simulink model "CLSfixedExample3"  (R2025b)
settings: Solver=FixedStepAuto  StartTime=0.0  StopTime=10  FixedStep=0.0005  RelTol=1e-3
undefined symbols (not defined in the file): AVI, cfg_length, CV1, CV2, LRI, pNode_length, pPath_length, PVARP, stepsize, URI, VRP
libraries: Libs x8, Libs_unified x3
(part 1 of 2)
settings Model: SimulationMode=accelerator  Creator=ball907  LastModifiedBy=rfen801
settings SolverCC: AutoInsertRateTranBlk=on
settings OptimizationCC: DefaultParameterBehavior=Inlined
settings ModelReferenceCC: EnableRefExpFcnMdlSchedulingChecks=on
settings RTWCC: Toolchain=Simulink Real-Time Toolchain  BuildConfiguration=Faster Runs  CodeExecutionProfiling=on

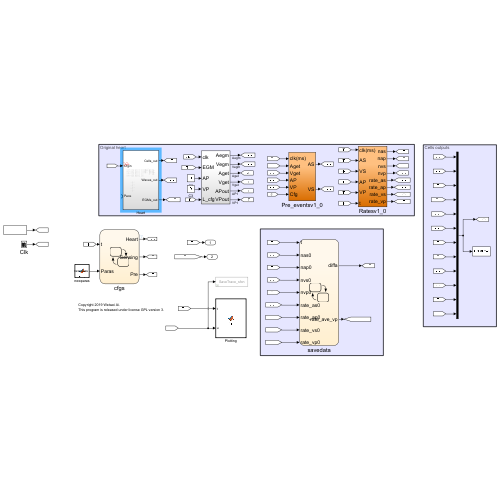
[thumbnail: Simulink's stored preview of the top-level diagram]
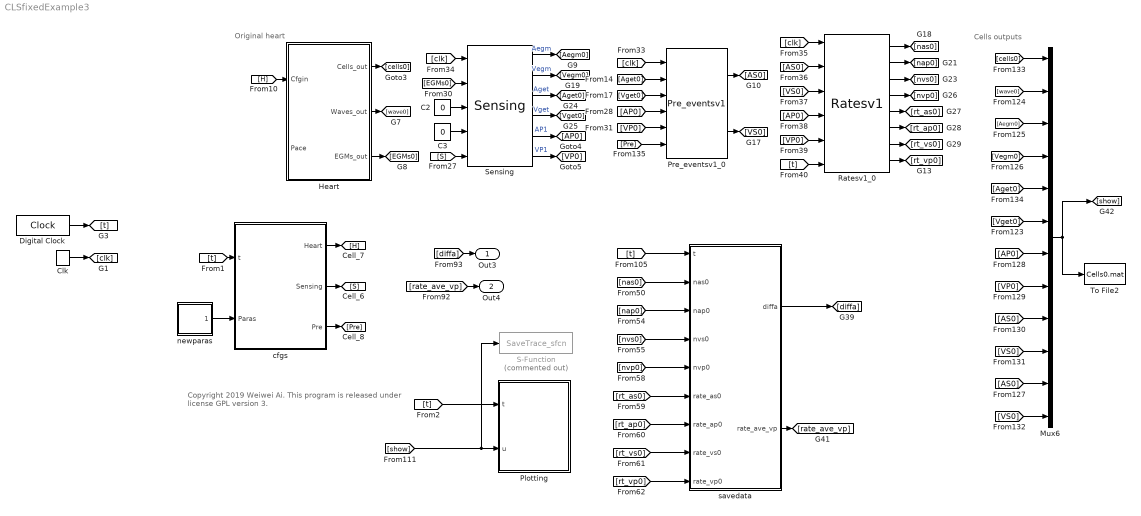
== system CLSfixedExample3 ==
  note: Cells outputs
  note: Copyright 2019 Weiwei Ai.
      | This program is released under license GPL version 3.
  note: Original heart
  C2 : Constant  Value=0
  C3 : Constant  Value=0
  Clk : DiscretePulseGenerator  PulseType=Time based  Period=1  PulseWidth=50
  Digital Clock : DigitalClock  SampleTime=stepsize
  Heart : Subsystem
  Mux6 : Mux  Inputs=12
  Plotting : MATLAB Function  TreatAsAtomicUnit=on  SystemSampleTime=stepsize*5
  Pre_eventsv1_0 : Libs_unified/Pre_eventsv1  SystemSampleTime=-1  VariantActivationTime=update diagram  EmptyChoice=off  PassThrough=off  PassThroughVariantControl=(default)  EmptyChoiceVariantControl=(default)  AllowFlexibleInterface=on  Latency=0  AutoFrameSizeCalculation=off
  Ratesv1_0 : Libs_unified/Ratesv1  SystemSampleTime=-1  VariantActivationTime=update diagram  EmptyChoice=off  PassThrough=off  PassThroughVariantControl=(default)  EmptyChoiceVariantControl=(default)  AllowFlexibleInterface=on  Latency=0  AutoFrameSizeCalculation=off
  S-Function : S-Function  Commented=on  FunctionName=SaveTrace_sfcn  Parameters=1  SFunctionDeploymentMode=off  EnableBusSupport=off
  Sensing : Libs_unified/Sensing  SystemSampleTime=-1  VariantActivationTime=update diagram  EmptyChoice=off  PassThrough=off  PassThroughVariantControl=(default)  EmptyChoiceVariantControl=(default)  AllowFlexibleInterface=on  Latency=0  AutoFrameSizeCalculation=off
  To File2 : ToFile  Filename=Cells0.mat  MatrixName=cells
      settings: Decimation=2
  cfgs : Stateflow chart  TreatAsAtomicUnit=on
  newparas : MATLAB Function  TreatAsAtomicUnit=on
  savedata : Stateflow chart  TreatAsAtomicUnit=on
  Out3 : Outport
  Out4 : Outport  Port=2
  wires:
  Sensing/6 -> [VP0]  "VP1"
  [VS0] -> Mux6/10
  [VS0] -> Ratesv1_0/3
  Pre_eventsv1_0/1 -> [AS0]
  [nap0] -> savedata/3(nap0)
  [VP0] -> Pre_eventsv1_0/5
  [AS0] -> Mux6/11
  Sensing/3 -> [Aget0]  "Aget"
  [rt_ap0] -> savedata/7(rate_ap0)
  C3/1 -> Sensing/4
  [AS0] -> Mux6/9
  Sensing/1 -> [Aegm0]  "Aegm"
  Ratesv1_0/4 -> [nvp0]
  [t] -> savedata/1(t)
  savedata/1(diffa) -> [diffa]
  Heart/3(EGMs_out) -> [EGMs0]
  [cells0] -> Mux6/1
  Pre_eventsv1_0/2 -> [VS0]
  Sensing/4 -> [Vget0]  "Vget"
  Ratesv1_0/5 -> [rt_as0]
  Ratesv1_0/3 -> [nvs0]
  [rt_vp0] -> savedata/9(rate_vp0)
  [rt_vs0] -> savedata/8(rate_vs0)
  [Aget0] -> Pre_eventsv1_0/2
  Sensing/5 -> [AP0]  "AP1"
  Ratesv1_0/1 -> [nas0]
  [diffa] -> Out3/1
  Heart/1(Cells_out) -> [cells0]
  Ratesv1_0/2 -> [nap0]
  [VP0] -> Mux6/8
  Mux6/1 -> [show], To File2/1
  [AS0] -> Ratesv1_0/2
  [AP0] -> Mux6/7
  [t] -> Ratesv1_0/6
  [Aegm0] -> Mux6/3
  [nvs0] -> savedata/4(nvs0)
  [Vget0] -> Mux6/6
  [rt_as0] -> savedata/6(rate_as0)
  [VS0] -> Mux6/12
  [AP0] -> Ratesv1_0/4
  Heart/2(Waves_out) -> [wave0]
  [clk] -> Ratesv1_0/1
  [clk] -> Pre_eventsv1_0/1
  [Pre] -> Pre_eventsv1_0/6
  [Vget0] -> Pre_eventsv1_0/3
  [wave0] -> Mux6/2
  [VP0] -> Ratesv1_0/5
  [AP0] -> Pre_eventsv1_0/4
  savedata/2(rate_ave_vp) -> [rate_ave_vp]
  C2/1 -> Sensing/3
  [S] -> Sensing/5
  [rate_ave_vp] -> Out4/1
  Ratesv1_0/7 -> [rt_vs0]
  [Vegm0] -> Mux6/4
  [clk] -> Sensing/1
  Ratesv1_0/8 -> [rt_vp0]
  [Aget0] -> Mux6/5
  ? -> ?
  [nas0] -> savedata/2(nas0)
  [EGMs0] -> Sensing/2
  Sensing/2 -> [Vegm0]  "Vegm"
  Ratesv1_0/6 -> [rt_ap0]
  [nvp0] -> savedata/5(nvp0)
  cfgs/2(Sensing) -> [S]
  cfgs/3(Pre) -> [Pre]
  newparas/1(newparas) -> cfgs/2(Paras)
  cfgs/1(Heart) -> [H]
  [t] -> cfgs/1(t)
  Digital Clock/1 -> [t]
  Clk/1 -> [clk]
  [show] -> S-Function/1, Plotting/2(u)
  [t] -> Plotting/1(t)
  [H] -> Heart/1(Cfgin)

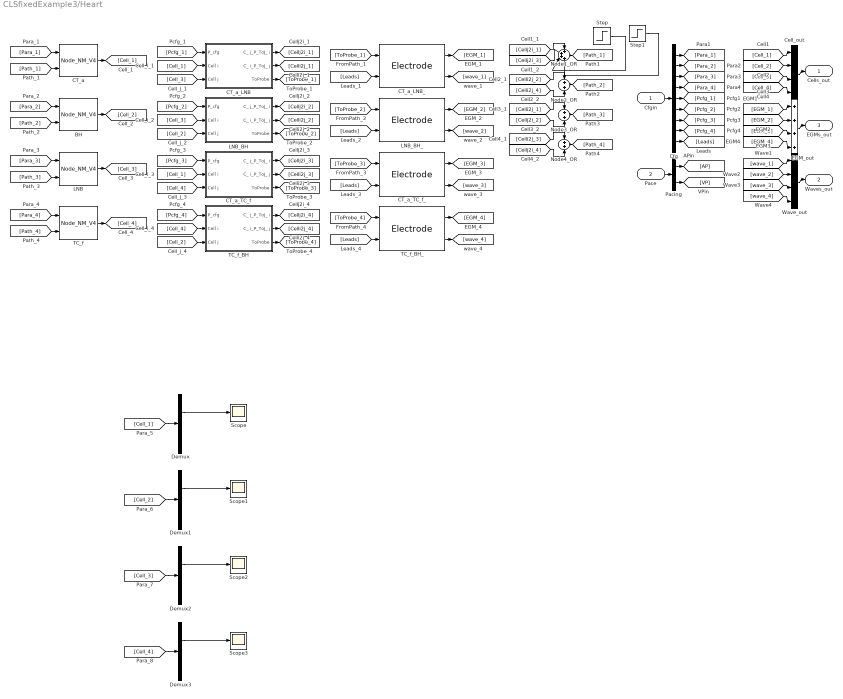
== system CLSfixedExample3/Heart ==
  Cfgin : Inport
  Pace : Inport  Port=2
  BH : Libs/Node_NM_V4  SystemSampleTime=-1  VariantActivationTime=update diagram  EmptyChoice=off  PassThrough=off  PassThroughVariantControl=(default)  EmptyChoiceVariantControl=(default)  AllowFlexibleInterface=on  Latency=0  AutoFrameSizeCalculation=off
  CT_a : Libs/Node_NM_V4  SystemSampleTime=-1  VariantActivationTime=update diagram  EmptyChoice=off  PassThrough=off  PassThroughVariantControl=(default)  EmptyChoiceVariantControl=(default)  AllowFlexibleInterface=on  Latency=0  AutoFrameSizeCalculation=off
  CT_a_LNB : Subsystem  AncestorBlock=Libs/Path_V3
  CT_a_LNB_ : Libs/Electrode  SystemSampleTime=-1  VariantActivationTime=update diagram  EmptyChoice=off  PassThrough=off  PassThroughVariantControl=(default)  EmptyChoiceVariantControl=(default)  AllowFlexibleInterface=on  Latency=0  AutoFrameSizeCalculation=off
  CT_a_TC_f : Subsystem  AncestorBlock=Libs/Path_V3
  CT_a_TC_f_ : Libs/Electrode  SystemSampleTime=-1  VariantActivationTime=update diagram  EmptyChoice=off  PassThrough=off  PassThroughVariantControl=(default)  EmptyChoiceVariantControl=(default)  AllowFlexibleInterface=on  Latency=0  AutoFrameSizeCalculation=off
  Cell_out : Mux
  Cfg : Demux  Outputs=[50,50,50,50,11,11,11,11,28]
  Demux{,1..3} (4 alike) : Demux  Outputs=5
  EGM_out : Sum  Inputs=4
  LNB : Libs/Node_NM_V4  SystemSampleTime=-1  VariantActivationTime=update diagram  EmptyChoice=off  PassThrough=off  PassThroughVariantControl=(default)  EmptyChoiceVariantControl=(default)  AllowFlexibleInterface=on  Latency=0  AutoFrameSizeCalculation=off
  LNB_BH : Subsystem  AncestorBlock=Libs/Path_V3
  LNB_BH_ : Libs/Electrode  SystemSampleTime=-1  VariantActivationTime=update diagram  EmptyChoice=off  PassThrough=off  PassThroughVariantControl=(default)  EmptyChoiceVariantControl=(default)  AllowFlexibleInterface=on  Latency=0  AutoFrameSizeCalculation=off
  Node1_OR : Sum  Inputs=4
  Node2_OR : Sum  Inputs=2
  Node3_OR : Sum  Inputs=2
  Node4_OR : Sum  Inputs=2
  Pacing : Demux  Outputs=2
  Scope{,1..3} (4 alike) : Scope
      Scope settings: ActiveDisplayYMinimum=-14.055953139718371  ActiveDisplayYMaximum=126.50357825746536
      Scope1 settings: ActiveDisplayYMinimum=-16.387499999999996  ActiveDisplayYMaximum=147.48749999999998
      Scope2 settings: ActiveDisplayYMinimum=-16.387499999999996  ActiveDisplayYMaximum=147.48749999999998  DataLoggingVariableName=ScopeData2
      Scope3 settings: ActiveDisplayYMinimum=-14.055953139718371  ActiveDisplayYMaximum=126.50357825746536  DataLoggingVariableName=ScopeData3
  Step : Step  Time=3.32  After=120  SampleTime=0
  Step1 : Step  Time=3.36  After=-120  SampleTime=0
  TC_f : Libs/Node_NM_V4  SystemSampleTime=-1  VariantActivationTime=update diagram  EmptyChoice=off  PassThrough=off  PassThroughVariantControl=(default)  EmptyChoiceVariantControl=(default)  AllowFlexibleInterface=on  Latency=0  AutoFrameSizeCalculation=off
  TC_f_BH : Subsystem  AncestorBlock=Libs/Path_V3
  TC_f_BH_ : Libs/Electrode  SystemSampleTime=-1  VariantActivationTime=update diagram  EmptyChoice=off  PassThrough=off  PassThroughVariantControl=(default)  EmptyChoiceVariantControl=(default)  AllowFlexibleInterface=on  Latency=0  AutoFrameSizeCalculation=off
  Wave_out : Mux
  Cells_out : Outport
  Waves_out : Outport  Port=2
  EGMs_out : Outport  Port=3
  wires:
  Demux1/2 -> Scope1/1
  [Cell_1] -> Demux/1
  [Cell_2] -> Demux1/1
  Demux/2 -> Scope/1
  [Cell_4] -> Demux3/1
  Demux3/2 -> Scope3/1
  [Cell_3] -> Demux2/1
  Demux2/2 -> Scope2/1
  Step1/1 -> Node1_OR/4
  Step/1 -> Node1_OR/3
  [wave_4] -> Wave_out/4
  [wave_3] -> Wave_out/3
  [wave_2] -> Wave_out/2
  [wave_1] -> Wave_out/1
  [EGM_4] -> EGM_out/4
  [EGM_3] -> EGM_out/3
  [EGM_2] -> EGM_out/2
  [EGM_1] -> EGM_out/1
  [Cell_4] -> Cell_out/4
  [Cell_3] -> Cell_out/3
  [Cell_2] -> Cell_out/2
  [Cell_1] -> Cell_out/1
  Wave_out/1 -> Waves_out/1
  EGM_out/1 -> EGMs_out/1
  Cell_out/1 -> Cells_out/1
  Pacing/2 -> [VP]
  Pacing/1 -> [AP]
  Cfg/9 -> [Leads]
  Cfg/8 -> [Pcfg_4]
  Cfg/7 -> [Pcfg_3]
  Cfg/6 -> [Pcfg_2]
  Cfg/5 -> [Pcfg_1]
  Cfg/4 -> [Para_4]
  Cfg/3 -> [Para_3]
  Cfg/2 -> [Para_2]
  Cfg/1 -> [Para_1]
  Pace/1 -> Pacing/1
  Cfgin/1 -> Cfg/1
  Node4_OR/1 -> [Path_4]
  [Cellj2i_4] -> Node4_OR/2
  [Celli2j_3] -> Node4_OR/1
  Node3_OR/1 -> [Path_3]
  [Cellj2i_2] -> Node3_OR/2
  [Celli2j_1] -> Node3_OR/1
  Node2_OR/1 -> [Path_2]
  [Celli2j_4] -> Node2_OR/2
  [Celli2j_2] -> Node2_OR/1
  Node1_OR/1 -> [Path_1]
  [Cellj2i_3] -> Node1_OR/2
  [Cellj2i_1] -> Node1_OR/1
  [Leads] -> TC_f_BH_/2
  [ToProbe_4] -> TC_f_BH_/1
  TC_f_BH_/2 -> [wave_4]
  TC_f_BH_/1 -> [EGM_4]
  [Leads] -> CT_a_TC_f_/2
  [ToProbe_3] -> CT_a_TC_f_/1
  CT_a_TC_f_/2 -> [wave_3]
  CT_a_TC_f_/1 -> [EGM_3]
  [Leads] -> LNB_BH_/2
  [ToProbe_2] -> LNB_BH_/1
  LNB_BH_/2 -> [wave_2]
  LNB_BH_/1 -> [EGM_2]
  [Leads] -> CT_a_LNB_/2
  [ToProbe_1] -> CT_a_LNB_/1
  CT_a_LNB_/2 -> [wave_1]
  CT_a_LNB_/1 -> [EGM_1]
  [Cell_2] -> TC_f_BH/3(Cell j)
  [Cell_4] -> TC_f_BH/2(Cell i)
  [Pcfg_4] -> TC_f_BH/1(P_cfg)
  TC_f_BH/3(ToProbe) -> [ToProbe_4]
  TC_f_BH/2(C_ i_P_ToJ_ j) -> [Celli2j_4]
  TC_f_BH/1(C_ j_P_ToJ_ i) -> [Cellj2i_4]
  [Cell_4] -> CT_a_TC_f/3(Cell j)
  [Cell_1] -> CT_a_TC_f/2(Cell i)
  [Pcfg_3] -> CT_a_TC_f/1(P_cfg)
  CT_a_TC_f/3(ToProbe) -> [ToProbe_3]
  CT_a_TC_f/2(C_ i_P_ToJ_ j) -> [Celli2j_3]
  CT_a_TC_f/1(C_ j_P_ToJ_ i) -> [Cellj2i_3]
  [Cell_2] -> LNB_BH/3(Cell j)
  [Cell_3] -> LNB_BH/2(Cell i)
  [Pcfg_2] -> LNB_BH/1(P_cfg)
  LNB_BH/3(ToProbe) -> [ToProbe_2]
  LNB_BH/2(C_ i_P_ToJ_ j) -> [Celli2j_2]
  LNB_BH/1(C_ j_P_ToJ_ i) -> [Cellj2i_2]
  [Cell_3] -> CT_a_LNB/3(Cell j)
  [Cell_1] -> CT_a_LNB/2(Cell i)
  [Pcfg_1] -> CT_a_LNB/1(P_cfg)
  CT_a_LNB/3(ToProbe) -> [ToProbe_1]
  CT_a_LNB/2(C_ i_P_ToJ_ j) -> [Celli2j_1]
  CT_a_LNB/1(C_ j_P_ToJ_ i) -> [Cellj2i_1]
  [Path_4] -> TC_f/2
  [Para_4] -> TC_f/1
  TC_f/1 -> [Cell_4]
  [Path_3] -> LNB/2
  [Para_3] -> LNB/1
  LNB/1 -> [Cell_3]
  [Path_2] -> BH/2
  [Para_2] -> BH/1
  BH/1 -> [Cell_2]
  [Path_1] -> CT_a/2
  [Para_1] -> CT_a/1
  CT_a/1 -> [Cell_1]

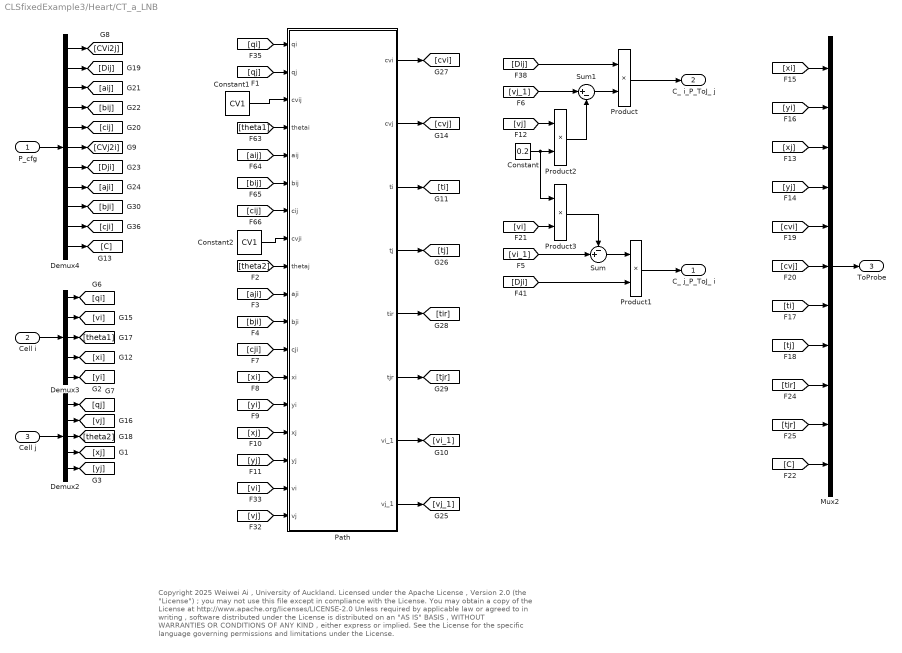
== system CLSfixedExample3/Heart/CT_a_LNB ==
  note: Copyright 2025 Weiwei Ai , University of Auckland.
      | Licensed under the Apache License , Version 2.0 (the "License") ;
      | you may not use this file except in compliance with the License.
      | You may obtain a copy of the License at
      | http://www.apache.org/licenses/LICENSE-2.0
      | Unless required by applicable law or agreed to in writing , software
      | distributed under the License is distributed on an "AS IS" BASIS ,
      | WITHOUT WARRANTIES OR CONDITIONS OF ANY KIND , either express or implied.
      | See the License for the specific language governing permissions and
      | limitations under the License.
  P_cfg : Inport
  Cell i : Inport  Port=2
  Cell j : Inport  Port=3
  Constant : Constant  Value=0.2
  Constant1 : Constant  Value=CV1
  Constant2 : Constant  Value=CV1
  Demux2 : Demux  Outputs=5
  Demux3 : Demux  Outputs=5
  Demux4 : Demux  Outputs=11
  Mux2 : Mux  Inputs=11
  Path : Stateflow chart  TreatAsAtomicUnit=on
  Product{,1..3} (4 alike) : Product  Inputs=**
  Sum : Sum  Inputs=-+|
  Sum1 : Sum  Inputs=|+-
  C_ j_P_ToJ_ i : Outport
  C_ i_P_ToJ_ j : Outport  Port=2
  ToProbe : Outport  Port=3
  wires:
  [vi] -> Product3/2
  [Dji] -> Product1/2
  [vi_1] -> Sum/2
  Product3/1 -> Sum/1
  Sum/1 -> Product1/1
  Constant/1 -> Product2/2, Product3/1
  Product2/1 -> Sum1/2
  [vj] -> Product2/1
  Sum1/1 -> Product/2
  [vj_1] -> Sum1/1
  Mux2/1 -> ToProbe/1
  [C] -> Mux2/11
  [tjr] -> Mux2/10
  [tj] -> Mux2/8
  [ti] -> Mux2/7
  [cvj] -> Mux2/6
  [tir] -> Mux2/9
  [cvi] -> Mux2/5
  [yj] -> Mux2/4
  [xj] -> Mux2/3
  [yi] -> Mux2/2
  [xi] -> Mux2/1
  Path/6(tjr) -> [tjr]
  Path/5(tir) -> [tir]
  Path/4(tj) -> [tj]
  Path/3(ti) -> [ti]
  Path/2(cvj) -> [cvj]
  Path/1(cvi) -> [cvi]
  Path/7(vi_1) -> [vi_1]
  Path/8(vj_1) -> [vj_1]
  [qj] -> Path/2(qj)
  Constant2/1 -> Path/8(cvji)
  [theta2] -> Path/9(thetaj)
  [aji] -> Path/10(aji)
  [bji] -> Path/11(bji)
  [cji] -> Path/12(cji)
  Demux4/6 -> [CVj2i]
  Demux4/7 -> [Dji]
  Demux4/8 -> [aji]
  Demux4/9 -> [bji]
  Demux4/10 -> [cji]
  Demux4/11 -> [C]
  Constant1/1 -> Path/3(cvij)
  [yj] -> Path/16(yj)
  [xj] -> Path/15(xj)
  [yi] -> Path/14(yi)
  [xi] -> Path/13(xi)
  Demux4/1 -> [CVi2j]
  Demux4/5 -> [cij]
  Demux4/4 -> [bij]
  Demux4/3 -> [aij]
  Demux4/2 -> [Dij]
  [cij] -> Path/7(cij)
  [bij] -> Path/6(bij)
  [aij] -> Path/5(aij)
  [theta1] -> Path/4(thetai)
  [Dij] -> Product/1
  Demux2/3 -> [theta2]
  Demux3/3 -> [theta1]
  [vj] -> Path/18(vj)
  Demux2/2 -> [vj]
  [vi] -> Path/17(vi)
  Demux3/2 -> [vi]
  Demux2/5 -> [yj]
  Demux2/4 -> [xj]
  Demux3/5 -> [yi]
  Demux3/4 -> [xi]
  Demux2/1 -> [qj]
  [qi] -> Path/1(qi)
  Demux3/1 -> [qi]
  Product1/1 -> C_ j_P_ToJ_ i/1
  Product/1 -> C_ i_P_ToJ_ j/1
  P_cfg/1 -> Demux4/1
  Cell j/1 -> Demux2/1
  Cell i/1 -> Demux3/1

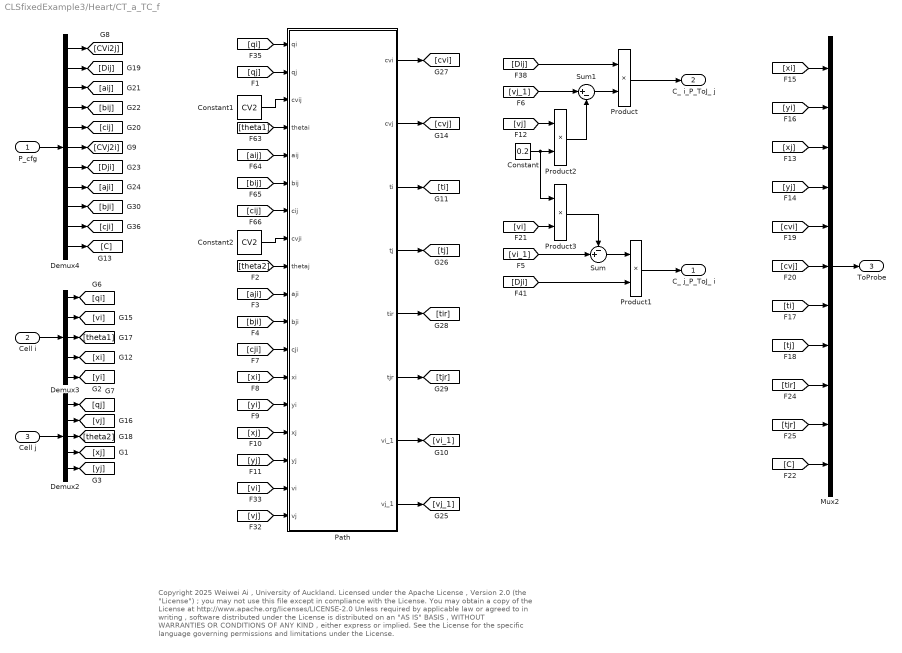
== system CLSfixedExample3/Heart/CT_a_TC_f ==
  note: Copyright 2025 Weiwei Ai , University of Auckland.
      | Licensed under the Apache License , Version 2.0 (the "License") ;
      | you may not use this file except in compliance with the License.
      | You may obtain a copy of the License at
      | http://www.apache.org/licenses/LICENSE-2.0
      | Unless required by applicable law or agreed to in writing , software
      | distributed under the License is distributed on an "AS IS" BASIS ,
      | WITHOUT WARRANTIES OR CONDITIONS OF ANY KIND , either express or implied.
      | See the License for the specific language governing permissions and
      | limitations under the License.
  P_cfg : Inport
  Cell i : Inport  Port=2
  Cell j : Inport  Port=3
  Constant : Constant  Value=0.2
  Constant1 : Constant  Value=CV2
  Constant2 : Constant  Value=CV2
  Demux2 : Demux  Outputs=5
  Demux3 : Demux  Outputs=5
  Demux4 : Demux  Outputs=11
  Mux2 : Mux  Inputs=11
  Path : Stateflow chart  TreatAsAtomicUnit=on
  Product{,1..3} (4 alike) : Product  Inputs=**
  Sum : Sum  Inputs=-+|
  Sum1 : Sum  Inputs=|+-
  C_ j_P_ToJ_ i : Outport
  C_ i_P_ToJ_ j : Outport  Port=2
  ToProbe : Outport  Port=3
  wires:
  [vi] -> Product3/2
  [Dji] -> Product1/2
  [vi_1] -> Sum/2
  Product3/1 -> Sum/1
  Sum/1 -> Product1/1
  Constant/1 -> Product2/2, Product3/1
  Product2/1 -> Sum1/2
  [vj] -> Product2/1
  Sum1/1 -> Product/2
  [vj_1] -> Sum1/1
  Mux2/1 -> ToProbe/1
  [C] -> Mux2/11
  [tjr] -> Mux2/10
  [tj] -> Mux2/8
  [ti] -> Mux2/7
  [cvj] -> Mux2/6
  [tir] -> Mux2/9
  [cvi] -> Mux2/5
  [yj] -> Mux2/4
  [xj] -> Mux2/3
  [yi] -> Mux2/2
  [xi] -> Mux2/1
  Path/6(tjr) -> [tjr]
  Path/5(tir) -> [tir]
  Path/4(tj) -> [tj]
  Path/3(ti) -> [ti]
  Path/2(cvj) -> [cvj]
  Path/1(cvi) -> [cvi]
  Path/7(vi_1) -> [vi_1]
  Path/8(vj_1) -> [vj_1]
  [qj] -> Path/2(qj)
  Constant2/1 -> Path/8(cvji)
  [theta2] -> Path/9(thetaj)
  [aji] -> Path/10(aji)
  [bji] -> Path/11(bji)
  [cji] -> Path/12(cji)
  Demux4/6 -> [CVj2i]
  Demux4/7 -> [Dji]
  Demux4/8 -> [aji]
  Demux4/9 -> [bji]
  Demux4/10 -> [cji]
  Demux4/11 -> [C]
  Constant1/1 -> Path/3(cvij)
  [yj] -> Path/16(yj)
  [xj] -> Path/15(xj)
  [yi] -> Path/14(yi)
  [xi] -> Path/13(xi)
  Demux4/1 -> [CVi2j]
  Demux4/5 -> [cij]
  Demux4/4 -> [bij]
  Demux4/3 -> [aij]
  Demux4/2 -> [Dij]
  [cij] -> Path/7(cij)
  [bij] -> Path/6(bij)
  [aij] -> Path/5(aij)
  [theta1] -> Path/4(thetai)
  [Dij] -> Product/1
  Demux2/3 -> [theta2]
  Demux3/3 -> [theta1]
  [vj] -> Path/18(vj)
  Demux2/2 -> [vj]
  [vi] -> Path/17(vi)
  Demux3/2 -> [vi]
  Demux2/5 -> [yj]
  Demux2/4 -> [xj]
  Demux3/5 -> [yi]
  Demux3/4 -> [xi]
  Demux2/1 -> [qj]
  [qi] -> Path/1(qi)
  Demux3/1 -> [qi]
  Product1/1 -> C_ j_P_ToJ_ i/1
  Product/1 -> C_ i_P_ToJ_ j/1
  P_cfg/1 -> Demux4/1
  Cell j/1 -> Demux2/1
  Cell i/1 -> Demux3/1

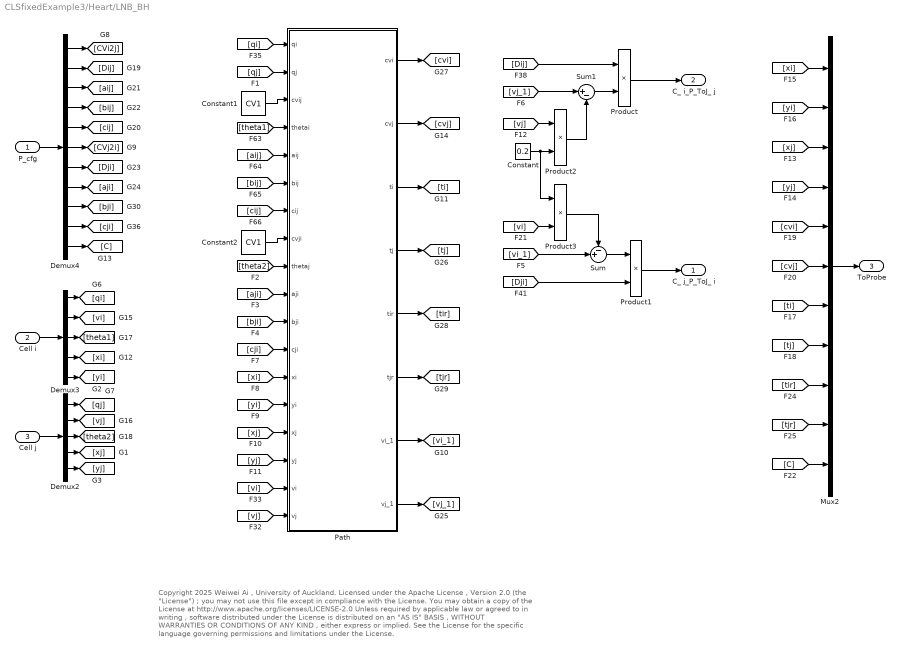
== system CLSfixedExample3/Heart/LNB_BH ==
  note: Copyright 2025 Weiwei Ai , University of Auckland.
      | Licensed under the Apache License , Version 2.0 (the "License") ;
      | you may not use this file except in compliance with the License.
      | You may obtain a copy of the License at
      | http://www.apache.org/licenses/LICENSE-2.0
      | Unless required by applicable law or agreed to in writing , software
      | distributed under the License is distributed on an "AS IS" BASIS ,
      | WITHOUT WARRANTIES OR CONDITIONS OF ANY KIND , either express or implied.
      | See the License for the specific language governing permissions and
      | limitations under the License.
  P_cfg : Inport
  Cell i : Inport  Port=2
  Cell j : Inport  Port=3
  Constant : Constant  Value=0.2
  Constant1 : Constant  Value=CV1
  Constant2 : Constant  Value=CV1
  Demux2 : Demux  Outputs=5
  Demux3 : Demux  Outputs=5
  Demux4 : Demux  Outputs=11
  Mux2 : Mux  Inputs=11
  Path : Stateflow chart  TreatAsAtomicUnit=on
  Product{,1..3} (4 alike) : Product  Inputs=**
  Sum : Sum  Inputs=-+|
  Sum1 : Sum  Inputs=|+-
  C_ j_P_ToJ_ i : Outport
  C_ i_P_ToJ_ j : Outport  Port=2
  ToProbe : Outport  Port=3
  wires:
  [vi] -> Product3/2
  [Dji] -> Product1/2
  [vi_1] -> Sum/2
  Product3/1 -> Sum/1
  Sum/1 -> Product1/1
  Constant/1 -> Product2/2, Product3/1
  Product2/1 -> Sum1/2
  [vj] -> Product2/1
  Sum1/1 -> Product/2
  [vj_1] -> Sum1/1
  Mux2/1 -> ToProbe/1
  [C] -> Mux2/11
  [tjr] -> Mux2/10
  [tj] -> Mux2/8
  [ti] -> Mux2/7
  [cvj] -> Mux2/6
  [tir] -> Mux2/9
  [cvi] -> Mux2/5
  [yj] -> Mux2/4
  [xj] -> Mux2/3
  [yi] -> Mux2/2
  [xi] -> Mux2/1
  Path/6(tjr) -> [tjr]
  Path/5(tir) -> [tir]
  Path/4(tj) -> [tj]
  Path/3(ti) -> [ti]
  Path/2(cvj) -> [cvj]
  Path/1(cvi) -> [cvi]
  Path/7(vi_1) -> [vi_1]
  Path/8(vj_1) -> [vj_1]
  [qj] -> Path/2(qj)
  Constant2/1 -> Path/8(cvji)
  [theta2] -> Path/9(thetaj)
  [aji] -> Path/10(aji)
  [bji] -> Path/11(bji)
  [cji] -> Path/12(cji)
  Demux4/6 -> [CVj2i]
  Demux4/7 -> [Dji]
  Demux4/8 -> [aji]
  Demux4/9 -> [bji]
  Demux4/10 -> [cji]
  Demux4/11 -> [C]
  Constant1/1 -> Path/3(cvij)
  [yj] -> Path/16(yj)
  [xj] -> Path/15(xj)
  [yi] -> Path/14(yi)
  [xi] -> Path/13(xi)
  Demux4/1 -> [CVi2j]
  Demux4/5 -> [cij]
  Demux4/4 -> [bij]
  Demux4/3 -> [aij]
  Demux4/2 -> [Dij]
  [cij] -> Path/7(cij)
  [bij] -> Path/6(bij)
  [aij] -> Path/5(aij)
  [theta1] -> Path/4(thetai)
  [Dij] -> Product/1
  Demux2/3 -> [theta2]
  Demux3/3 -> [theta1]
  [vj] -> Path/18(vj)
  Demux2/2 -> [vj]
  [vi] -> Path/17(vi)
  Demux3/2 -> [vi]
  Demux2/5 -> [yj]
  Demux2/4 -> [xj]
  Demux3/5 -> [yi]
  Demux3/4 -> [xi]
  Demux2/1 -> [qj]
  [qi] -> Path/1(qi)
  Demux3/1 -> [qi]
  Product1/1 -> C_ j_P_ToJ_ i/1
  Product/1 -> C_ i_P_ToJ_ j/1
  P_cfg/1 -> Demux4/1
  Cell j/1 -> Demux2/1
  Cell i/1 -> Demux3/1

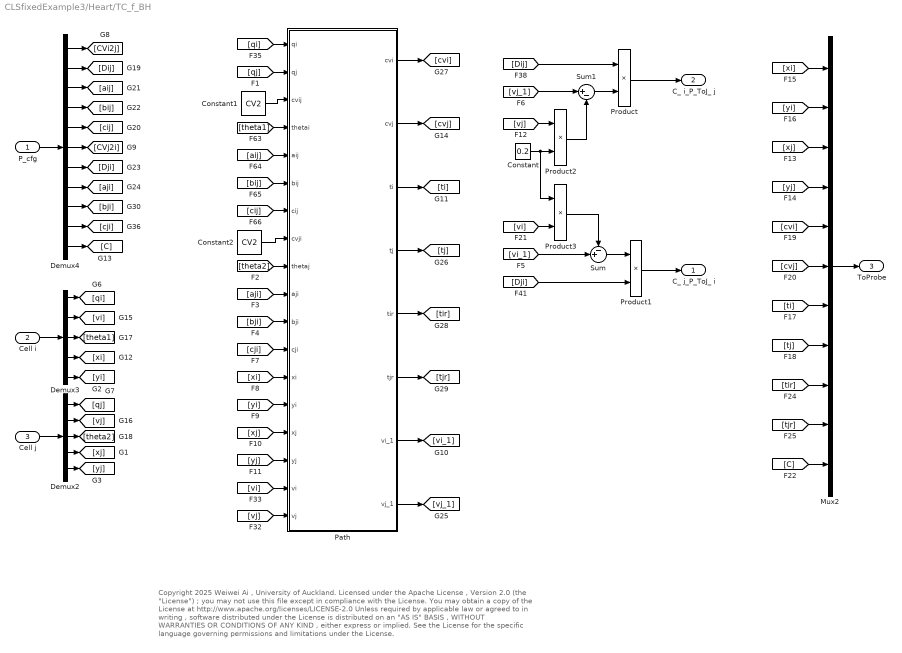
== system CLSfixedExample3/Heart/TC_f_BH ==
  note: Copyright 2025 Weiwei Ai , University of Auckland.
      | Licensed under the Apache License , Version 2.0 (the "License") ;
      | you may not use this file except in compliance with the License.
      | You may obtain a copy of the License at
      | http://www.apache.org/licenses/LICENSE-2.0
      | Unless required by applicable law or agreed to in writing , software
      | distributed under the License is distributed on an "AS IS" BASIS ,
      | WITHOUT WARRANTIES OR CONDITIONS OF ANY KIND , either express or implied.
      | See the License for the specific language governing permissions and
      | limitations under the License.
  P_cfg : Inport
  Cell i : Inport  Port=2
  Cell j : Inport  Port=3
  Constant : Constant  Value=0.2
  Constant1 : Constant  Value=CV2
  Constant2 : Constant  Value=CV2
  Demux2 : Demux  Outputs=5
  Demux3 : Demux  Outputs=5
  Demux4 : Demux  Outputs=11
  Mux2 : Mux  Inputs=11
  Path : Stateflow chart  TreatAsAtomicUnit=on
  Product{,1..3} (4 alike) : Product  Inputs=**
  Sum : Sum  Inputs=-+|
  Sum1 : Sum  Inputs=|+-
  C_ j_P_ToJ_ i : Outport
  C_ i_P_ToJ_ j : Outport  Port=2
  ToProbe : Outport  Port=3
  wires:
  [vi] -> Product3/2
  [Dji] -> Product1/2
  [vi_1] -> Sum/2
  Product3/1 -> Sum/1
  Sum/1 -> Product1/1
  Constant/1 -> Product2/2, Product3/1
  Product2/1 -> Sum1/2
  [vj] -> Product2/1
  Sum1/1 -> Product/2
  [vj_1] -> Sum1/1
  Mux2/1 -> ToProbe/1
  [C] -> Mux2/11
  [tjr] -> Mux2/10
  [tj] -> Mux2/8
  [ti] -> Mux2/7
  [cvj] -> Mux2/6
  [tir] -> Mux2/9
  [cvi] -> Mux2/5
  [yj] -> Mux2/4
  [xj] -> Mux2/3
  [yi] -> Mux2/2
  [xi] -> Mux2/1
  Path/6(tjr) -> [tjr]
  Path/5(tir) -> [tir]
  Path/4(tj) -> [tj]
  Path/3(ti) -> [ti]
  Path/2(cvj) -> [cvj]
  Path/1(cvi) -> [cvi]
  Path/7(vi_1) -> [vi_1]
  Path/8(vj_1) -> [vj_1]
  [qj] -> Path/2(qj)
  Constant2/1 -> Path/8(cvji)
  [theta2] -> Path/9(thetaj)
  [aji] -> Path/10(aji)
  [bji] -> Path/11(bji)
  [cji] -> Path/12(cji)
  Demux4/6 -> [CVj2i]
  Demux4/7 -> [Dji]
  Demux4/8 -> [aji]
  Demux4/9 -> [bji]
  Demux4/10 -> [cji]
  Demux4/11 -> [C]
  Constant1/1 -> Path/3(cvij)
  [yj] -> Path/16(yj)
  [xj] -> Path/15(xj)
  [yi] -> Path/14(yi)
  [xi] -> Path/13(xi)
  Demux4/1 -> [CVi2j]
  Demux4/5 -> [cij]
  Demux4/4 -> [bij]
  Demux4/3 -> [aij]
  Demux4/2 -> [Dij]
  [cij] -> Path/7(cij)
  [bij] -> Path/6(bij)
  [aij] -> Path/5(aij)
  [theta1] -> Path/4(thetai)
  [Dij] -> Product/1
  Demux2/3 -> [theta2]
  Demux3/3 -> [theta1]
  [vj] -> Path/18(vj)
  Demux2/2 -> [vj]
  [vi] -> Path/17(vi)
  Demux3/2 -> [vi]
  Demux2/5 -> [yj]
  Demux2/4 -> [xj]
  Demux3/5 -> [yi]
  Demux3/4 -> [xi]
  Demux2/1 -> [qj]
  [qi] -> Path/1(qi)
  Demux3/1 -> [qi]
  Product1/1 -> C_ j_P_ToJ_ i/1
  Product/1 -> C_ i_P_ToJ_ j/1
  P_cfg/1 -> Demux4/1
  Cell j/1 -> Demux2/1
  Cell i/1 -> Demux3/1

== stateflow chart CLSfixedExample3/savedata ==
  settings: executeAtInitialization=1
  state termi
  state difa
  state Ini
  difa -> termi [order 1] : [rate_ave_a0>=60]/{coder.extrinsic('assignin');diffa=rate_ave_a1-rate_ave_a0;assignin('base', 'diffa', diffa);}
  (default) -> Ini : {rate_ave_vp=0; diffa=0;}
  Ini -> difa : [t>=29998]{coder.extrinsic('assignin','mean');...
      | assignin('base', 'nas0', nas0);assignin('base', 'nap0', nap0);assignin('base', 'nvs0', nvs0);assignin('base', 'nvp0', nvp0);...
      | assignin('base', 'rate_as0', rate_as0);assignin('base', 'rate_ap0', rate_ap0);assignin('base', 'rate_vs0', rate_vs0);assignin('base', 'rate_vp0', rate_vp0);...
      | rate_ave_vp=mean(rate_vp0(2,1:nvp0));assignin('base', 'rate_ave_vp', rate_ave_vp);...
      | rate_ave_a1=0;rate_ave_a0=0;rate_ave_a0=mean(rate_as0(2,1:nas0));rate_ave_a1=zeros(size(rate_ave_a0),like=rate_ave_a0);}
  difa -> termi [order 2] : [rate_ave_a0<60]/{coder.extrinsic('assignin');diffa=rate_ave_a1-60;assignin('base', 'diffa', diffa);}
  data: t input; nas0 input; nap0 input; nvs0 input; nvp0 input; rate_as0 input; rate_ap0 input; rate_vs0 input; rate_vp0 input; diffa output double; rate_ave_vp output double; rate_ave_a0 local double; rate_ave_a1 local double

== stateflow chart CLSfixedExample3/Heart/TC_f_BH/Path ==
  settings: updateMethod=DISCRETE
  state Wave
    state Relay_i [parallel]
      settings: executionOrder=8
      state Relay
        en: tj_1=0;
        du: tj_1=temporalCount(sec);
        vj_1=vbi(floor(tj_1)+1);
        ex: tj_1=0;
      state Idle
        en:
        vj_1=0;
      Wave.Relay_i.Idle -> Wave.Relay_i.Relay : Reach_j
      (default) -> Wave.Relay_i.Idle
      Wave.Relay_i.Relay -> Wave.Relay_i.Idle : [qj>=2 || j_1==0 ]
    state Cell_i_1 [parallel]
      settings: executionOrder=5
      state Activation
      state Rest
        en:
        i_1=0;
      Wave.Cell_i_1.Rest -> Wave.Cell_i_1.Activation : Reach_i
      Wave.Cell_i_1.Activation -> Wave.Cell_i_1.Rest [order 1] : [after(tbj,sec)]
      (default) -> Wave.Cell_i_1.Rest
      Wave.Cell_i_1.Activation -> Wave.Cell_i_1.Rest [order 2] : Go_j
    state Relay_j [parallel]
      settings: executionOrder=7
      state Relay
        en: ti_1=0;
        du: ti_1=temporalCount(sec);
        vi_1=vbj(floor(ti_1)+1);
        ex: ti_1=0;
      state Idle
        en:
        vi_1=0;
      Wave.Relay_j.Idle -> Wave.Relay_j.Relay : Reach_i
      (default) -> Wave.Relay_j.Idle
      Wave.Relay_j.Relay -> Wave.Relay_j.Idle : [qi>=2 || i_1==0 ]
    state Cell_j_1 [parallel]
      settings: executionOrder=6
      state Activation
      state Rest
        en:
        j_1=0;
      note: 1.
      Wave.Cell_j_1.Rest -> Wave.Cell_j_1.Activation : Reach_j
      Wave.Cell_j_1.Activation -> Wave.Cell_j_1.Rest [order 1] : [after(tbi,sec)]
      (default) -> Wave.Cell_j_1.Rest
      Wave.Cell_j_1.Activation -> Wave.Cell_j_1.Rest [order 2] : Go_i
    state End_j [parallel]
      settings: executionOrder=2
      state End_j_Idle
      state Go
        en: tj=0;
        du: tj=temporalCount(sec);
        ex: tj=0;
      note: 5
      state Ready
      note: 2.
      state BlockedByNeighbour
      Wave.End_j.Go -> Wave.End_j.End_j_Idle [order 2] : [Meet || mul==0]
      Wave.End_j.Go -> Wave.End_j.End_j_Idle [order 1] : [tj>=Tj && mul==1]
          | /{mul=mul-1;i_1=1; Reach_i;}
      (default) -> Wave.End_j.End_j_Idle
      Wave.End_j.End_j_Idle -> Wave.End_j.Ready [order 1] : [qj==2 && j_1==0]
      Wave.End_j.Ready -> Wave.End_j.Go [order 2] : [qj==3 && j_1==0]
          | /{ cvj=thetafcn(cvji,thetaj,aji,bji,cji);
          | Tj=l/cvj; mul=mul+1; Go_j;}
      Wave.End_j.End_j_Idle -> Wave.End_j.BlockedByNeighbour [order 2] : [qj==2 && j_1==1]
      Wave.End_j.Ready -> Wave.End_j.BlockedByNeighbour [order 1] : [cvji==0 || (qj==3 && j_1==1)]{tj=0;}
      Wave.End_j.BlockedByNeighbour -> Wave.End_j.End_j_Idle : [qj==0]
    state End_i [parallel]
      settings: executionOrder=1
      state Go
        en:ti=0;
        du: ti=temporalCount(sec);
        ex: ti=0;
      state End_i_Idle
      note: 4
      state Ready
      note: 2.
      note: 7
      state BlockedByNeighbour
      Wave.End_i.Go -> Wave.End_i.End_i_Idle [order 2] : [cvi*ti+cvj*tj>=l && mul==2]/
          | { mul=0; Meet;}
      Wave.End_i.Go -> Wave.End_i.End_i_Idle [order 1] : [ti>=Ti && mul==1]
          | /{mul=mul-1; j_1=1; Reach_j;}
      (default) -> Wave.End_i.End_i_Idle
      Wave.End_i.End_i_Idle -> Wave.End_i.Ready [order 1] : [qi==2 && i_1==0]
      Wave.End_i.Ready -> Wave.End_i.Go [order 2] : [qi==3 && i_1==0]
          | /{ cvi=thetafcn(cvij,thetai,aij,bij,cij);
          | Ti=l/cvi; mul=mul+1;Go_i; }
      Wave.End_i.End_i_Idle -> Wave.End_i.BlockedByNeighbour [order 2] : [qi==2 && i_1==1]
      Wave.End_i.Ready -> Wave.End_i.BlockedByNeighbour [order 1] : [cvij==0 || (qi==3 && i_1==1)]{ti=0;}
      Wave.End_i.BlockedByNeighbour -> Wave.End_i.End_i_Idle : [qi==0]
    state Buffer_i [parallel]
      settings: executionOrder=3
      state Idle
      note: 6
      state Buffer_i
        en: tbi=0;
        du: tbi=temporalCount(sec);
        vbi(floor(tbi)+1)=vi;
      (default) -> Wave.Buffer_i.Idle
      Wave.Buffer_i.Idle -> Wave.Buffer_i.Buffer_i : Go_i
      Wave.Buffer_i.Buffer_i -> Wave.Buffer_i.Idle [order 1] : [qi<3]
      Wave.Buffer_i.Buffer_i -> Wave.Buffer_i.Idle [order 2] : Meet
      Wave.Buffer_i.Buffer_i -> Wave.Buffer_i.Idle [order 3] : [tbi>=599]
    note: 3
    state Buffer_j [parallel]
      settings: executionOrder=4
      state Idle
      state Buffer_i
        en: tbj=0;
        du: tbj=temporalCount(sec);
        vbj(floor(tbj)+1)=vj;
      (default) -> Wave.Buffer_j.Idle
      Wave.Buffer_j.Idle -> Wave.Buffer_j.Buffer_i : Go_j
      Wave.Buffer_j.Buffer_i -> Wave.Buffer_j.Idle [order 1] : [qj<3]
      Wave.Buffer_j.Buffer_i -> Wave.Buffer_j.Idle [order 2] : Meet
      Wave.Buffer_j.Buffer_i -> Wave.Buffer_j.Idle [order 3] : [tbj>=599]
    state End_i_Fade [parallel]
      settings: executionOrder=10
      state End_i_Idle
      state End_i_re
        du: tir=temporalCount(sec);
      End_i_re -> Wave.End_i_Fade.End_i_Idle [order 1] : [cvi*tir+cvj*tjr>=l && tjr~=0]/{Meet_r;tir=0;tjr=0;}
      End_i_re -> Wave.End_i_Fade.End_i_Idle [order 2] : [cvi*tir+cvj*tjr>=l&& tjr==0]/{tir=0;}
      (default) -> Wave.End_i_Fade.End_i_Idle
      Wave.End_i_Fade.End_i_Idle -> End_i_re : cell_i_r
    state End_j_Fade [parallel]
      settings: executionOrder=12
      state End_j_Idle
      state End_j_re
        du: tjr=temporalCount(sec);
      End_j_re -> Wave.End_j_Fade.End_j_Idle [order 1] : [cvi*tir+cvj*tjr>=l&& tir==0]/{tjr=0;}
      End_j_re -> Wave.End_j_Fade.End_j_Idle [order 2] : Meet_r
      (default) -> Wave.End_j_Fade.End_j_Idle
      Wave.End_j_Fade.End_j_Idle -> End_j_re : cell_j_r
    state Celll_j_Re [parallel]
      settings: executionOrder=9
      state Re
      state De
      Wave.Celll_j_Re.De -> Wave.Celll_j_Re.Re : [qj==0]/{cell_j_r;}
      Wave.Celll_j_Re.Re -> Wave.Celll_j_Re.De : [qj==3]
      (default) -> Wave.Celll_j_Re.Re
    state Celll_i_Re [parallel]
      settings: executionOrder=11
      state Re
      state De
      Wave.Celll_i_Re.De -> Wave.Celll_i_Re.Re : [qi==0]/{cell_i_r;}
      Wave.Celll_i_Re.Re -> Wave.Celll_i_Re.De : [qi==3]
      (default) -> Wave.Celll_i_Re.Re
    note: 1. The Cell_j_1 will be released if it has been resting or another AP from Cell_i starts travelling;.
    note: 2. Cell_i start to repolarize before the activation either reaches Cell_j or meets the activation from Cell_j, which happens when the APD is short or/and the path is long, e.g., premature depolarization.
        | In this case, the path would ignore all following activation before the premature activation reaches Cell_j or meets the activation from Cell_j.
  note: 3. Assume that the APD<=600 ms; If the APD>600, it would be truncated; Store the action potential of q3 until it goes back to repolarization or meets the other one.
      | 4. j_1=1; and Reach_j must occur at the same time to block Go_j immediately;
      | 5. mul==0 to make sure the transition to take in case Meet event is missed
      | 6. qi<3 instead of qi==0 to avoid where qi==0 is missed due to the stimulation timing and the simulation step;
      | 7. when cv=0, no propagation.
  (default) -> Wave : /{l=sqrt((xj-xi)^2+(yj-yi)^2);
      | cvi=cvij;
      | cvj=cvji;
      | Ti=1/cvi;
      | Tj=1/cvj;
      | ti=0;
      | tj=0;
      | ti_1=0;
      | tj_1=0;
      | i_1=0;
      | j_1=0;
      | vi_1=0;
      | vj_1=0;
      | tir=0;
      | tjr=0;
      | tbi=0;
      | tbj=0;
      | vbi=zeros(1,600);
      | vbj=zeros(1,600);
      | mul=0;
      | }
  data: cvin function_input double; thetain function_input double; ain function_input double; bin function_input double; cin function_input double; cvout function_output double; cvi output double; cvj output double; ti output double; qi input; qj input; ti_1 local double; tj_1 local double; cvij input; thetai input; aij input; bij input; cij input; cvji input; thetaj input; aji input; bji input; cji input; xi input; yi input; xj input; yj input; tj output; tir output; tjr output; i_1 local; j_1 local; vi_1 output; vj_1 output; l local; tbi local; tbj local; vbi local; vbj local; vi input; vj input; Ti local double; Tj local double; mul local
  events: Reach_i local FUNCTION_CALL_EVENT; Reach_j local FUNCTION_CALL_EVENT; Go_i local FUNCTION_CALL_EVENT; Go_j local FUNCTION_CALL_EVENT; Meet local FUNCTION_CALL_EVENT; Meet_r local FUNCTION_CALL_EVENT; cell_i_r local FUNCTION_CALL_EVENT; cell_j_r local FUNCTION_CALL_EVENT
  function cvout = thetafcn(cvin,thetain,ain,bin,cin):
    | function cvout = thetafcn(cvin,thetain,ain,bin,cin)
    | %#codegen
    | %Rate dependent factor
    | ftheta=1/(ain*exp(bin*thetain)+(1-ain)*exp(-cin*thetain));
    | cvout=cvin*ftheta;
    | end

== stateflow chart CLSfixedExample3/Heart/CT_a_LNB/Path ==
  settings: updateMethod=DISCRETE
  state Wave
    state Relay_i [parallel]
      settings: executionOrder=8
      state Relay
        en: tj_1=0;
        du: tj_1=temporalCount(sec);
        vj_1=vbi(floor(tj_1)+1);
        ex: tj_1=0;
      state Idle
        en:
        vj_1=0;
      Wave.Relay_i.Idle -> Wave.Relay_i.Relay : Reach_j
      (default) -> Wave.Relay_i.Idle
      Wave.Relay_i.Relay -> Wave.Relay_i.Idle : [qj>=2 || j_1==0 ]
    state Cell_i_1 [parallel]
      settings: executionOrder=5
      state Activation
      state Rest
        en:
        i_1=0;
      Wave.Cell_i_1.Rest -> Wave.Cell_i_1.Activation : Reach_i
      Wave.Cell_i_1.Activation -> Wave.Cell_i_1.Rest [order 1] : [after(tbj,sec)]
      (default) -> Wave.Cell_i_1.Rest
      Wave.Cell_i_1.Activation -> Wave.Cell_i_1.Rest [order 2] : Go_j
    state Relay_j [parallel]
      settings: executionOrder=7
      state Relay
        en: ti_1=0;
        du: ti_1=temporalCount(sec);
        vi_1=vbj(floor(ti_1)+1);
        ex: ti_1=0;
      state Idle
        en:
        vi_1=0;
      Wave.Relay_j.Idle -> Wave.Relay_j.Relay : Reach_i
      (default) -> Wave.Relay_j.Idle
      Wave.Relay_j.Relay -> Wave.Relay_j.Idle : [qi>=2 || i_1==0 ]
    state Cell_j_1 [parallel]
      settings: executionOrder=6
      state Activation
      state Rest
        en:
        j_1=0;
      note: 1.
      Wave.Cell_j_1.Rest -> Wave.Cell_j_1.Activation : Reach_j
      Wave.Cell_j_1.Activation -> Wave.Cell_j_1.Rest [order 1] : [after(tbi,sec)]
      (default) -> Wave.Cell_j_1.Rest
      Wave.Cell_j_1.Activation -> Wave.Cell_j_1.Rest [order 2] : Go_i
    state End_j [parallel]
      settings: executionOrder=2
      state End_j_Idle
      state Go
        en: tj=0;
        du: tj=temporalCount(sec);
        ex: tj=0;
      note: 5
      state Ready
      note: 2.
      state BlockedByNeighbour
      Wave.End_j.Go -> Wave.End_j.End_j_Idle [order 2] : [Meet || mul==0]
      Wave.End_j.Go -> Wave.End_j.End_j_Idle [order 1] : [tj>=Tj && mul==1]
          | /{mul=mul-1;i_1=1; Reach_i;}
      (default) -> Wave.End_j.End_j_Idle
      Wave.End_j.End_j_Idle -> Wave.End_j.Ready [order 1] : [qj==2 && j_1==0]
      Wave.End_j.Ready -> Wave.End_j.Go [order 2] : [qj==3 && j_1==0]
          | /{ cvj=thetafcn(cvji,thetaj,aji,bji,cji);
          | Tj=l/cvj; mul=mul+1; Go_j;}
      Wave.End_j.End_j_Idle -> Wave.End_j.BlockedByNeighbour [order 2] : [qj==2 && j_1==1]
      Wave.End_j.Ready -> Wave.End_j.BlockedByNeighbour [order 1] : [cvji==0 || (qj==3 && j_1==1)]{tj=0;}
      Wave.End_j.BlockedByNeighbour -> Wave.End_j.End_j_Idle : [qj==0]
    state End_i [parallel]
      settings: executionOrder=1
      state Go
        en:ti=0;
        du: ti=temporalCount(sec);
        ex: ti=0;
      state End_i_Idle
      note: 4
      state Ready
      note: 2.
      note: 7
      state BlockedByNeighbour
      Wave.End_i.Go -> Wave.End_i.End_i_Idle [order 2] : [cvi*ti+cvj*tj>=l && mul==2]/
          | { mul=0; Meet;}
      Wave.End_i.Go -> Wave.End_i.End_i_Idle [order 1] : [ti>=Ti && mul==1]
          | /{mul=mul-1; j_1=1; Reach_j;}
      (default) -> Wave.End_i.End_i_Idle
      Wave.End_i.End_i_Idle -> Wave.End_i.Ready [order 1] : [qi==2 && i_1==0]
      Wave.End_i.Ready -> Wave.End_i.Go [order 2] : [qi==3 && i_1==0]
          | /{ cvi=thetafcn(cvij,thetai,aij,bij,cij);
          | Ti=l/cvi; mul=mul+1;Go_i; }
      Wave.End_i.End_i_Idle -> Wave.End_i.BlockedByNeighbour [order 2] : [qi==2 && i_1==1]
      Wave.End_i.Ready -> Wave.End_i.BlockedByNeighbour [order 1] : [cvij==0 || (qi==3 && i_1==1)]{ti=0;}
      Wave.End_i.BlockedByNeighbour -> Wave.End_i.End_i_Idle : [qi==0]
    state Buffer_i [parallel]
      settings: executionOrder=3
      state Idle
      note: 6
      state Buffer_i
        en: tbi=0;
        du: tbi=temporalCount(sec);
        vbi(floor(tbi)+1)=vi;
      (default) -> Wave.Buffer_i.Idle
      Wave.Buffer_i.Idle -> Wave.Buffer_i.Buffer_i : Go_i
      Wave.Buffer_i.Buffer_i -> Wave.Buffer_i.Idle [order 1] : [qi<3]
      Wave.Buffer_i.Buffer_i -> Wave.Buffer_i.Idle [order 2] : Meet
      Wave.Buffer_i.Buffer_i -> Wave.Buffer_i.Idle [order 3] : [tbi>=599]
    note: 3
    state Buffer_j [parallel]
      settings: executionOrder=4
      state Idle
      state Buffer_i
        en: tbj=0;
        du: tbj=temporalCount(sec);
        vbj(floor(tbj)+1)=vj;
      (default) -> Wave.Buffer_j.Idle
      Wave.Buffer_j.Idle -> Wave.Buffer_j.Buffer_i : Go_j
      Wave.Buffer_j.Buffer_i -> Wave.Buffer_j.Idle [order 1] : [qj<3]
      Wave.Buffer_j.Buffer_i -> Wave.Buffer_j.Idle [order 2] : Meet
      Wave.Buffer_j.Buffer_i -> Wave.Buffer_j.Idle [order 3] : [tbj>=599]
    state End_i_Fade [parallel]
      settings: executionOrder=10
      state End_i_Idle
      state End_i_re
        du: tir=temporalCount(sec);
      End_i_re -> Wave.End_i_Fade.End_i_Idle [order 1] : [cvi*tir+cvj*tjr>=l && tjr~=0]/{Meet_r;tir=0;tjr=0;}
      End_i_re -> Wave.End_i_Fade.End_i_Idle [order 2] : [cvi*tir+cvj*tjr>=l&& tjr==0]/{tir=0;}
      (default) -> Wave.End_i_Fade.End_i_Idle
      Wave.End_i_Fade.End_i_Idle -> End_i_re : cell_i_r
    state End_j_Fade [parallel]
      settings: executionOrder=12
      state End_j_Idle
      state End_j_re
        du: tjr=temporalCount(sec);
      End_j_re -> Wave.End_j_Fade.End_j_Idle [order 1] : [cvi*tir+cvj*tjr>=l&& tir==0]/{tjr=0;}
      End_j_re -> Wave.End_j_Fade.End_j_Idle [order 2] : Meet_r
      (default) -> Wave.End_j_Fade.End_j_Idle
      Wave.End_j_Fade.End_j_Idle -> End_j_re : cell_j_r
    state Celll_j_Re [parallel]
      settings: executionOrder=9
      state Re
      state De
      Wave.Celll_j_Re.De -> Wave.Celll_j_Re.Re : [qj==0]/{cell_j_r;}
      Wave.Celll_j_Re.Re -> Wave.Celll_j_Re.De : [qj==3]
      (default) -> Wave.Celll_j_Re.Re
    state Celll_i_Re [parallel]
      settings: executionOrder=11
      state Re
      state De
      Wave.Celll_i_Re.De -> Wave.Celll_i_Re.Re : [qi==0]/{cell_i_r;}
      Wave.Celll_i_Re.Re -> Wave.Celll_i_Re.De : [qi==3]
      (default) -> Wave.Celll_i_Re.Re
    note: 1. The Cell_j_1 will be released if it has been resting or another AP from Cell_i starts travelling;.
    note: 2. Cell_i start to repolarize before the activation either reaches Cell_j or meets the activation from Cell_j, which happens when the APD is short or/and the path is long, e.g., premature depolarization.
        | In this case, the path would ignore all following activation before the premature activation reaches Cell_j or meets the activation from Cell_j.
  note: 3. Assume that the APD<=600 ms; If the APD>600, it would be truncated; Store the action potential of q3 until it goes back to repolarization or meets the other one.
      | 4. j_1=1; and Reach_j must occur at the same time to block Go_j immediately;
      | 5. mul==0 to make sure the transition to take in case Meet event is missed
      | 6. qi<3 instead of qi==0 to avoid where qi==0 is missed due to the stimulation timing and the simulation step;
      | 7. when cv=0, no propagation.
  (default) -> Wave : /{l=sqrt((xj-xi)^2+(yj-yi)^2);
      | cvi=cvij;
      | cvj=cvji;
      | Ti=1/cvi;
      | Tj=1/cvj;
      | ti=0;
      | tj=0;
      | ti_1=0;
      | tj_1=0;
      | i_1=0;
      | j_1=0;
      | vi_1=0;
      | vj_1=0;
      | tir=0;
      | tjr=0;
      | tbi=0;
      | tbj=0;
      | vbi=zeros(1,600);
      | vbj=zeros(1,600);
      | mul=0;
      | }
  data: cvin function_input double; thetain function_input double; ain function_input double; bin function_input double; cin function_input double; cvout function_output double; cvi output double; cvj output double; ti output double; qi input; qj input; ti_1 local double; tj_1 local double; cvij input; thetai input; aij input; bij input; cij input; cvji input; thetaj input; aji input; bji input; cji input; xi input; yi input; xj input; yj input; tj output; tir output; tjr output; i_1 local; j_1 local; vi_1 output; vj_1 output; l local; tbi local; tbj local; vbi local; vbj local; vi input; vj input; Ti local double; Tj local double; mul local
  events: Reach_i local FUNCTION_CALL_EVENT; Reach_j local FUNCTION_CALL_EVENT; Go_i local FUNCTION_CALL_EVENT; Go_j local FUNCTION_CALL_EVENT; Meet local FUNCTION_CALL_EVENT; Meet_r local FUNCTION_CALL_EVENT; cell_i_r local FUNCTION_CALL_EVENT; cell_j_r local FUNCTION_CALL_EVENT
  function cvout = thetafcn(cvin,thetain,ain,bin,cin):
    | function cvout = thetafcn(cvin,thetain,ain,bin,cin)
    | %#codegen
    | %Rate dependent factor
    | ftheta=1/(ain*exp(bin*thetain)+(1-ain)*exp(-cin*thetain));
    | cvout=cvin*ftheta;
    | end

== stateflow chart CLSfixedExample3/cfgs ==
  settings: executeAtInitialization=1
  state Ini
  state wait
  Ini -> wait : [t>800]{pUpdate(Paras);}
  (default) -> Ini : {Sensing=Scfgf;[Pre]=Precfg;...
      |  [Heart] =LoadInit;}
  data: Scfg function_output; Preout function_output; LRI parameter; AVI parameter; VRP parameter; URI parameter; PVARP parameter; Parasin function_input; pNode_length parameter; pPath_length parameter; Hcfg function_output; cfg_length parameter; Heart output; Sensing output; t input; Paras input; Pre output
  function Scfg= Scfgf:
    | function Scfg= Scfgf
    | 
    | %% desired
    | xa=1;
    | xc=0.05;
    | xc1=0.1;
    | xd=1;
    | xe=0.1;
    | avd=100;
    | vad=100;
    | uni_a=1;
    | Sens_a=0.6;
    | Amp_ap=500;
    | uni_v=1;
    | Sens_v=2.8;
    | Amp_vp=500;
    | 
    | Scfg=[xa xc xc1 xd xe avd vad uni_a Sens_a Amp_ap uni_v Sens_v Amp_vp]';
    | 
    | end
  function Preout = Precfg:
    | function Preout = Precfg
    | % 
    | % LRI=1000;
    | % AVI=170;
    | % URI=500;
    | % VRP=230;
    | % PVARP=250;
    | Preout=[VRP PVARP];
    | 
    | end
  function pUpdate(Parasin):
    | %% Get the index of the parameter
    | function pUpdate(Parasin)
    | %#codegen
    | coder.extrinsic('evalin');
    | coder.extrinsic('assignin');
    | Nodein=zeros(1,pNode_length); % The total number of cell cfg ports
    | Nodein=evalin('base', 'pNode');
    | Pathin=zeros(1,pPath_length); % The total number of path cfg ports
    | Pathin=evalin('base', 'pPath');
    | for n=1:pNode_length
    |     m=Nodein(n);
    |     Heart(m)=Parasin(n);
    | end
    | 
    | for n=1:pPath_length
    |     m=Pathin(n);
    |     nn=n+length(Nodein);
    |     Heart(m)=Parasin(nn);
    | end
    | 
    | assignin('base', 'Params', Parasin);
    | 
    | end
  function Hcfg   = LoadInit:
    | function Hcfg   = LoadInit
    | %#codegen
    | coder.extrinsic('evalin');
    | Hcfg1=zeros(1,cfg_length); % The total number of cfg ports
    | Hcfg1=evalin('base', 'cfgdata');
    | Hcfg=Hcfg1';
    | end

== matlab function CLSfixedExample3/Plotting ==
  data: t input; u input
function fcn(t,u)
%coder.extrinsic('evalin')
coder.extrinsic('updateGUIplots')
fun = 'updateGUIplots';
updateGUIplots(t,u)
%feval(fun,t,u)
end

== stateflow chart CLSfixedExample3/Heart/LNB_BH/Path ==
  settings: updateMethod=DISCRETE
  state Wave
    state Relay_i [parallel]
      settings: executionOrder=8
      state Relay
        en: tj_1=0;
        du: tj_1=temporalCount(sec);
        vj_1=vbi(floor(tj_1)+1);
        ex: tj_1=0;
      state Idle
        en:
        vj_1=0;
      Wave.Relay_i.Idle -> Wave.Relay_i.Relay : Reach_j
      (default) -> Wave.Relay_i.Idle
      Wave.Relay_i.Relay -> Wave.Relay_i.Idle : [qj>=2 || j_1==0 ]
    state Cell_i_1 [parallel]
      settings: executionOrder=5
      state Activation
      state Rest
        en:
        i_1=0;
      Wave.Cell_i_1.Rest -> Wave.Cell_i_1.Activation : Reach_i
      Wave.Cell_i_1.Activation -> Wave.Cell_i_1.Rest [order 1] : [after(tbj,sec)]
      (default) -> Wave.Cell_i_1.Rest
      Wave.Cell_i_1.Activation -> Wave.Cell_i_1.Rest [order 2] : Go_j
    state Relay_j [parallel]
      settings: executionOrder=7
      state Relay
        en: ti_1=0;
        du: ti_1=temporalCount(sec);
        vi_1=vbj(floor(ti_1)+1);
        ex: ti_1=0;
      state Idle
        en:
        vi_1=0;
      Wave.Relay_j.Idle -> Wave.Relay_j.Relay : Reach_i
      (default) -> Wave.Relay_j.Idle
      Wave.Relay_j.Relay -> Wave.Relay_j.Idle : [qi>=2 || i_1==0 ]
    state Cell_j_1 [parallel]
      settings: executionOrder=6
      state Activation
      state Rest
        en:
        j_1=0;
      note: 1.
      Wave.Cell_j_1.Rest -> Wave.Cell_j_1.Activation : Reach_j
      Wave.Cell_j_1.Activation -> Wave.Cell_j_1.Rest [order 1] : [after(tbi,sec)]
      (default) -> Wave.Cell_j_1.Rest
      Wave.Cell_j_1.Activation -> Wave.Cell_j_1.Rest [order 2] : Go_i
    state End_j [parallel]
      settings: executionOrder=2
      state End_j_Idle
      state Go
        en: tj=0;
        du: tj=temporalCount(sec);
        ex: tj=0;
      note: 5
      state Ready
      note: 2.
      state BlockedByNeighbour
      Wave.End_j.Go -> Wave.End_j.End_j_Idle [order 2] : [Meet || mul==0]
      Wave.End_j.Go -> Wave.End_j.End_j_Idle [order 1] : [tj>=Tj && mul==1]
          | /{mul=mul-1;i_1=1; Reach_i;}
      (default) -> Wave.End_j.End_j_Idle
      Wave.End_j.End_j_Idle -> Wave.End_j.Ready [order 1] : [qj==2 && j_1==0]
      Wave.End_j.Ready -> Wave.End_j.Go [order 2] : [qj==3 && j_1==0]
          | /{ cvj=thetafcn(cvji,thetaj,aji,bji,cji);
          | Tj=l/cvj; mul=mul+1; Go_j;}
      Wave.End_j.End_j_Idle -> Wave.End_j.BlockedByNeighbour [order 2] : [qj==2 && j_1==1]
      Wave.End_j.Ready -> Wave.End_j.BlockedByNeighbour [order 1] : [cvji==0 || (qj==3 && j_1==1)]{tj=0;}
      Wave.End_j.BlockedByNeighbour -> Wave.End_j.End_j_Idle : [qj==0]
    state End_i [parallel]
      settings: executionOrder=1
      state Go
        en:ti=0;
        du: ti=temporalCount(sec);
        ex: ti=0;
      state End_i_Idle
      note: 4
      state Ready
      note: 2.
      note: 7
      state BlockedByNeighbour
      Wave.End_i.Go -> Wave.End_i.End_i_Idle [order 2] : [cvi*ti+cvj*tj>=l && mul==2]/
          | { mul=0; Meet;}
      Wave.End_i.Go -> Wave.End_i.End_i_Idle [order 1] : [ti>=Ti && mul==1]
          | /{mul=mul-1; j_1=1; Reach_j;}
      (default) -> Wave.End_i.End_i_Idle
      Wave.End_i.End_i_Idle -> Wave.End_i.Ready [order 1] : [qi==2 && i_1==0]
      Wave.End_i.Ready -> Wave.End_i.Go [order 2] : [qi==3 && i_1==0]
          | /{ cvi=thetafcn(cvij,thetai,aij,bij,cij);
          | Ti=l/cvi; mul=mul+1;Go_i; }
      Wave.End_i.End_i_Idle -> Wave.End_i.BlockedByNeighbour [order 2] : [qi==2 && i_1==1]
      Wave.End_i.Ready -> Wave.End_i.BlockedByNeighbour [order 1] : [cvij==0 || (qi==3 && i_1==1)]{ti=0;}
      Wave.End_i.BlockedByNeighbour -> Wave.End_i.End_i_Idle : [qi==0]
    state Buffer_i [parallel]
      settings: executionOrder=3
      state Idle
      note: 6
      state Buffer_i
        en: tbi=0;
        du: tbi=temporalCount(sec);
        vbi(floor(tbi)+1)=vi;
      (default) -> Wave.Buffer_i.Idle
      Wave.Buffer_i.Idle -> Wave.Buffer_i.Buffer_i : Go_i
      Wave.Buffer_i.Buffer_i -> Wave.Buffer_i.Idle [order 1] : [qi<3]
      Wave.Buffer_i.Buffer_i -> Wave.Buffer_i.Idle [order 2] : Meet
      Wave.Buffer_i.Buffer_i -> Wave.Buffer_i.Idle [order 3] : [tbi>=599]
    note: 3
    state Buffer_j [parallel]
      settings: executionOrder=4
      state Idle
      state Buffer_i
        en: tbj=0;
        du: tbj=temporalCount(sec);
        vbj(floor(tbj)+1)=vj;
      (default) -> Wave.Buffer_j.Idle
      Wave.Buffer_j.Idle -> Wave.Buffer_j.Buffer_i : Go_j
      Wave.Buffer_j.Buffer_i -> Wave.Buffer_j.Idle [order 1] : [qj<3]
      Wave.Buffer_j.Buffer_i -> Wave.Buffer_j.Idle [order 2] : Meet
      Wave.Buffer_j.Buffer_i -> Wave.Buffer_j.Idle [order 3] : [tbj>=599]
    state End_i_Fade [parallel]
      settings: executionOrder=10
      state End_i_Idle
      state End_i_re
        du: tir=temporalCount(sec);
      End_i_re -> Wave.End_i_Fade.End_i_Idle [order 1] : [cvi*tir+cvj*tjr>=l && tjr~=0]/{Meet_r;tir=0;tjr=0;}
      End_i_re -> Wave.End_i_Fade.End_i_Idle [order 2] : [cvi*tir+cvj*tjr>=l&& tjr==0]/{tir=0;}
      (default) -> Wave.End_i_Fade.End_i_Idle
      Wave.End_i_Fade.End_i_Idle -> End_i_re : cell_i_r
    state End_j_Fade [parallel]
      settings: executionOrder=12
      state End_j_Idle
      state End_j_re
        du: tjr=temporalCount(sec);
      End_j_re -> Wave.End_j_Fade.End_j_Idle [order 1] : [cvi*tir+cvj*tjr>=l&& tir==0]/{tjr=0;}
      End_j_re -> Wave.End_j_Fade.End_j_Idle [order 2] : Meet_r
      (default) -> Wave.End_j_Fade.End_j_Idle
      Wave.End_j_Fade.End_j_Idle -> End_j_re : cell_j_r
    state Celll_j_Re [parallel]
      settings: executionOrder=9
      state Re
      state De
      Wave.Celll_j_Re.De -> Wave.Celll_j_Re.Re : [qj==0]/{cell_j_r;}
      Wave.Celll_j_Re.Re -> Wave.Celll_j_Re.De : [qj==3]
      (default) -> Wave.Celll_j_Re.Re
    state Celll_i_Re [parallel]
      settings: executionOrder=11
      state Re
      state De
      Wave.Celll_i_Re.De -> Wave.Celll_i_Re.Re : [qi==0]/{cell_i_r;}
      Wave.Celll_i_Re.Re -> Wave.Celll_i_Re.De : [qi==3]
      (default) -> Wave.Celll_i_Re.Re
    note: 1. The Cell_j_1 will be released if it has been resting or another AP from Cell_i starts travelling;.
    note: 2. Cell_i start to repolarize before the activation either reaches Cell_j or meets the activation from Cell_j, which happens when the APD is short or/and the path is long, e.g., premature depolarization.
        | In this case, the path would ignore all following activation before the premature activation reaches Cell_j or meets the activation from Cell_j.
  note: 3. Assume that the APD<=600 ms; If the APD>600, it would be truncated; Store the action potential of q3 until it goes back to repolarization or meets the other one.
      | 4. j_1=1; and Reach_j must occur at the same time to block Go_j immediately;
      | 5. mul==0 to make sure the transition to take in case Meet event is missed
      | 6. qi<3 instead of qi==0 to avoid where qi==0 is missed due to the stimulation timing and the simulation step;
      | 7. when cv=0, no propagation.
  (default) -> Wave : /{l=sqrt((xj-xi)^2+(yj-yi)^2);
      | cvi=cvij;
      | cvj=cvji;
      | Ti=1/cvi;
      | Tj=1/cvj;
      | ti=0;
      | tj=0;
      | ti_1=0;
      | tj_1=0;
      | i_1=0;
      | j_1=0;
      | vi_1=0;
      | vj_1=0;
      | tir=0;
      | tjr=0;
      | tbi=0;
      | tbj=0;
      | vbi=zeros(1,600);
      | vbj=zeros(1,600);
      | mul=0;
      | }
  data: cvin function_input double; thetain function_input double; ain function_input double; bin function_input double; cin function_input double; cvout function_output double; cvi output double; cvj output double; ti output double; qi input; qj input; ti_1 local double; tj_1 local double; cvij input; thetai input; aij input; bij input; cij input; cvji input; thetaj input; aji input; bji input; cji input; xi input; yi input; xj input; yj input; tj output; tir output; tjr output; i_1 local; j_1 local; vi_1 output; vj_1 output; l local; tbi local; tbj local; vbi local; vbj local; vi input; vj input; Ti local double; Tj local double; mul local
  events: Reach_i local FUNCTION_CALL_EVENT; Reach_j local FUNCTION_CALL_EVENT; Go_i local FUNCTION_CALL_EVENT; Go_j local FUNCTION_CALL_EVENT; Meet local FUNCTION_CALL_EVENT; Meet_r local FUNCTION_CALL_EVENT; cell_i_r local FUNCTION_CALL_EVENT; cell_j_r local FUNCTION_CALL_EVENT
  function cvout = thetafcn(cvin,thetain,ain,bin,cin):
    | function cvout = thetafcn(cvin,thetain,ain,bin,cin)
    | %#codegen
    | %Rate dependent factor
    | ftheta=1/(ain*exp(bin*thetain)+(1-ain)*exp(-cin*thetain));
    | cvout=cvin*ftheta;
    | end

== matlab function CLSfixedExample3/newparas ==
  data: newparas output; paras_length parameter

function newparas= auto(paras_length)

coder.extrinsic('evalin');
%par_length = evalin('base','paras_length')
newparas=zeros(1,paras_length); % The total number of cell cfg ports
newparas=evalin('base', 'pp');

end
